simulink model "QubeServo3Pendulum_Workspace"  (R2023a)
settings: Solver=ode4  StartTime=0.0  StopTime=inf  FixedStep=1/1000  RelTol=1e-3  EnableMultiTasking=on
model workspace (MAT data in the model file):
  Jp = 0.000133128
  Jr = 0.000228791666667
  Jr_stall = 1
  Jt = 1.31452806e-08
  Lp = 0.129
  Rm = 7.5
  bp = 3e-05
  bpp = 5e-05
  bpr = 0.000425
  br = 2.15e-05
  br_stall = 100
  brp = 0
  brr = 0.0005
  g = 9.81
  km = 0.0422
  kr = 0.0005
  kt = 0.0422
  l = 0.0645
  mp = 0.024
  mr = 0.095
  r = 0.085
libraries: quarc_library x6, simulink x6, simulink_extras x2
settings Model: SimulationMode=external  ExtModeTrigDuration=10000  Creator=mbohra  LastModifiedBy=mbohra
settings SolverCC: AlgebraicLoopSolver=TrustRegion  PositivePriorityOrder=on
settings DataIOCC: ReturnWorkspaceOutputs=off
settings OptimizationCC: ReuseModelBlockBuffer=off
settings DebuggingCC: UnconnectedInputMsg=warning  UnconnectedOutputMsg=warning  UnconnectedLineMsg=warning  ArithmeticOperatorsInVariantConditions=warning
settings ModelReferenceCC: EnableRefExpFcnMdlSchedulingChecks=on
settings SFSimCC: SimUseLocalCustomCode=off  CustomCodeUndefinedFunction=UseInterfaceOnly
settings RTWCC: Description=QUARC Win64 Target Using Toolchain  SystemTargetFile=quarc_win64.tlc  TemplateMakefile=quarc_default_tmf  RTWUseLocalCustomCode=off  Toolchain=QUARC win64 | nmake (64-bit Windows)  BuildConfiguration=Faster Runs  DLArmComputeVersion=19.05
settings CodeAppCC: StateflowObjectComments=on
settings STFCustomTargetCC: SystemTargetFile=quarc_win64.tlc
settings GRTTargetCC: ParMdlRefBuildCompliant=off  CompOptLevelCompliant=off  CombineOutputUpdateFcns=off  MatFileLogging=off  CPPClassGenCompliant=off  GRTInterface=on  ExtMode=on  ExtModeMexFile=quarc_comm
settings ConfigComp: CovMetricSettings=dswe

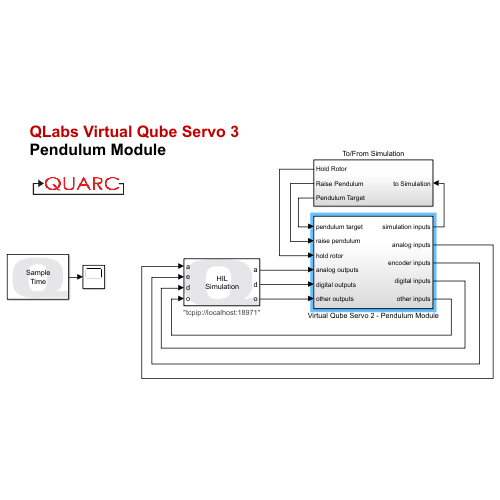
[thumbnail: Simulink's stored preview of the top-level diagram]
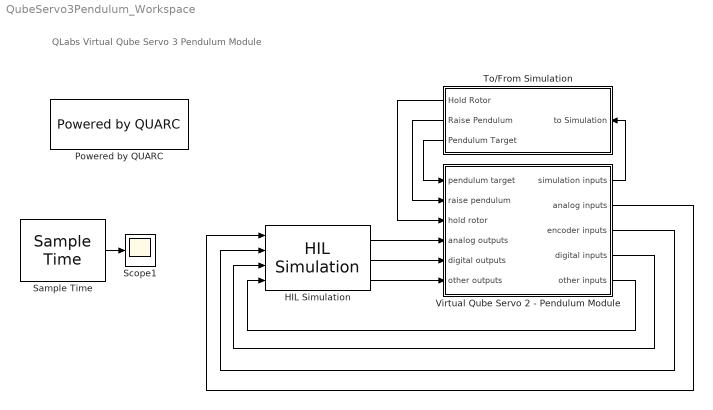
== system QubeServo3Pendulum_Workspace ==
  note: QLabs Virtual Qube Servo 3
      | Pendulum Module
  HIL Simulation : quarc_library/Data Acquisition/Generic/Configuration/HIL Simulation  uri_source=Specify via dialog (do not evaluate)  uri=tcpip://localhost:18971  board_type=qube_servo3_usb  board_id=0  sample_time=qc_get_step_size  active=on  num_clocks=1  num_interrupts=0  num_analog_inputs=1  num_analog_outputs=1  initial_analog=[]  num_digital_io=0  num_digital_inputs=3  num_digital_outputs=1  initial_digital=[]  num_encoder_inputs=2  num_pwm_outputs=0  initial_pwm=[]  other_inputs=[14000]  other_outputs=[11000:11002]  initial_other=[]  integer_get_property_codes=[]  double_get_property_codes=[]  string_get_property_codes=[]  integer_set_property_codes=[]  double_set_property_codes=[]  string_set_property_codes=[]  initial_integer_properties=0  initial_double_properties=0  max_string_property=80  use_variable_size_strings=off
      settings: AttributesFormatString="\"tcpip://localhost:18971\""  SourceProductName=QUARC Targets
  Powered by QUARC : quarc_library/Logos/Powered by QUARC
  Sample Time : quarc_library/Sources/Time/Sample Time  Priority=-99  sample_time=qc_get_step_size
  Scope1 : Scope
  To/From Simulation : Subsystem
  Virtual Qube Servo 2 - Pendulum Module : Subsystem
  wires:
  Sample Time/1 -> Scope1/1
  Virtual Qube Servo 2 - Pendulum Module/1(simulation inputs) -> To/From Simulation/1(to Simulation)
  HIL Simulation/1 -> Virtual Qube Servo 2 - Pendulum Module/4(analog outputs)
  HIL Simulation/2 -> Virtual Qube Servo 2 - Pendulum Module/5(digital outputs)
  Virtual Qube Servo 2 - Pendulum Module/2(analog inputs) -> HIL Simulation/1
  Virtual Qube Servo 2 - Pendulum Module/5(other inputs) -> HIL Simulation/4
  Virtual Qube Servo 2 - Pendulum Module/3(encoder inputs) -> HIL Simulation/2
  Virtual Qube Servo 2 - Pendulum Module/4(digital inputs) -> HIL Simulation/3
  To/From Simulation/2(Raise Pendulum) -> Virtual Qube Servo 2 - Pendulum Module/2(raise pendulum)
  To/From Simulation/1(Hold Rotor) -> Virtual Qube Servo 2 - Pendulum Module/3(hold rotor)
  HIL Simulation/3 -> Virtual Qube Servo 2 - Pendulum Module/6(other outputs)
  To/From Simulation/3(Pendulum Target) -> Virtual Qube Servo 2 - Pendulum Module/1(pendulum target)

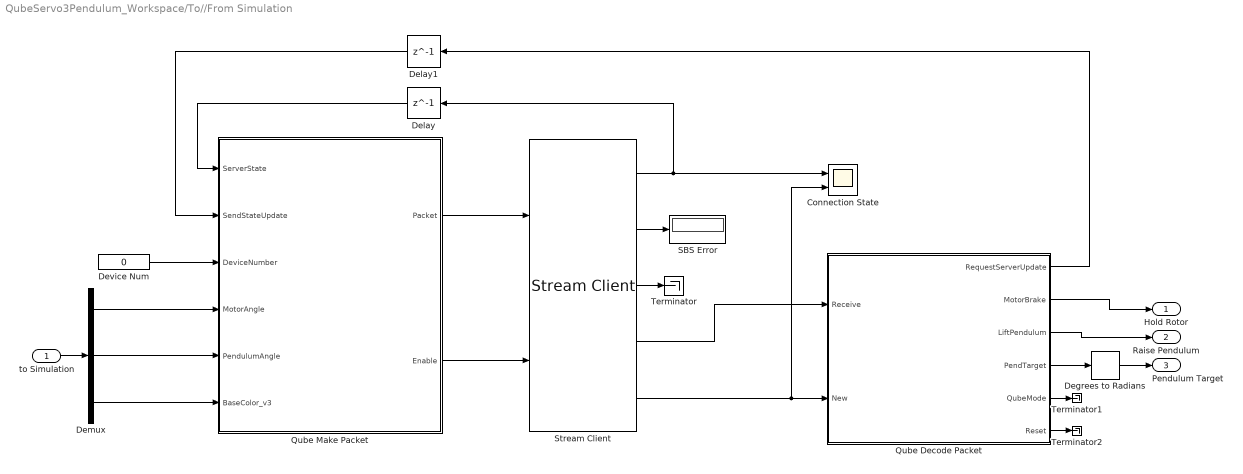
== system QubeServo3Pendulum_Workspace/To//From Simulation ==
  to Simulation : Inport
  "Connection State " : Scope  NumInputPorts=2
  Degrees to Radians : simulink_extras/Transformations/Degrees to Radians
  Delay : Delay  DelayLength=1
  Delay1 : Delay  DelayLength=1
  Demux : Demux  Outputs=[1,1,3]
  Device Num : Constant  Value=0
  Qube Decode Packet : MATLAB Function  TreatAsAtomicUnit=on
  Qube Make Packet : MATLAB Function  TreatAsAtomicUnit=on
  SBS Error : Display
  Stream Client : quarc_library/Communications/Basic/Stream Client  uri_source=Specify via dialog (do not evaluate)  uri=tcpip://localhost:18000?nagle='off'  send_buffer_size=65537  receive_buffer_size=65537  byte_order=little endian (Intel - LSB first)  optimization=Minimum latency  send_options=Send all data  receive_options=Receive all data  default_value=[0]  sample_time=qc_get_step_size  active=off  implementation=Use blocking I/O in a separate thread  send_fifo_size=3  receive_fifo_size=3  send_priority=0  receive_priority=0  send_dimensions=on  receive_dimensions=on  max_dimensions=65537  data_type=uint8  type_expr=BusObject
      settings: AttributesFormatString="\"tcpip://localhost:18000?nagle='off'\""
  Terminator : Terminator
  Terminator1 : Terminator
  Terminator2 : Terminator
  Hold Rotor : Outport  VectorParamsAs1DForOutWhenUnconnected=off
  Raise Pendulum : Outport  Port=2  VectorParamsAs1DForOutWhenUnconnected=off
  Pendulum Target : Outport  Port=3  VectorParamsAs1DForOutWhenUnconnected=off
  wires:
  Qube Make Packet/1(Packet) -> Stream Client/1
  Qube Make Packet/2(Enable) -> Stream Client/2
  Stream Client/2 -> SBS Error/1
  Demux/3 -> Qube Make Packet/6(BaseColor_v3)
  Qube Decode Packet/3(LiftPendulum) -> Raise Pendulum/1
  Delay/1 -> Qube Make Packet/1(ServerState)
  Stream Client/1 -> Delay/1, "Connection State "/1
  Stream Client/3 -> Terminator/1
  Qube Decode Packet/2(MotorBrake) -> Hold Rotor/1
  Delay1/1 -> Qube Make Packet/2(SendStateUpdate)
  Device Num/1 -> Qube Make Packet/3(DeviceNumber)
  Stream Client/5 -> "Connection State "/2, Qube Decode Packet/2(New)
  Demux/1 -> Qube Make Packet/4(MotorAngle)
  Qube Decode Packet/1(RequestServerUpdate) -> Delay1/1
  Stream Client/4 -> Qube Decode Packet/1(Receive)
  Demux/2 -> Qube Make Packet/5(PendulumAngle)
  to Simulation/1 -> Demux/1
  Qube Decode Packet/5(QubeMode) -> Terminator1/1
  Qube Decode Packet/6(Reset) -> Terminator2/1
  Qube Decode Packet/4(PendTarget) -> Degrees to Radians/1
  Degrees to Radians/1 -> Pendulum Target/1

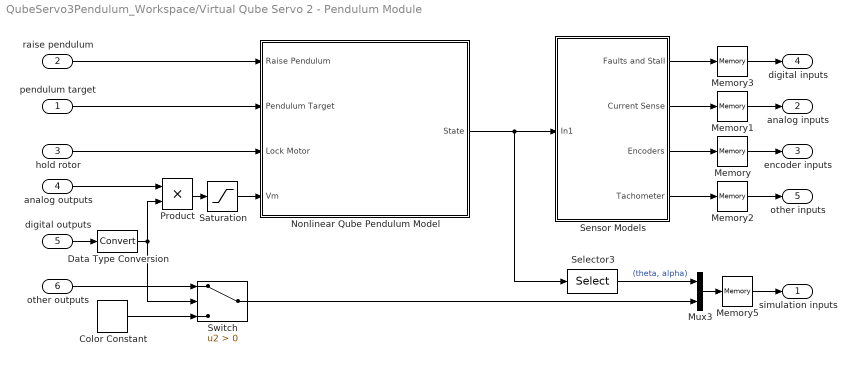
== system QubeServo3Pendulum_Workspace/Virtual Qube Servo 2 - Pendulum Module ==
  pendulum target : Inport
  raise pendulum : Inport  Port=2
  hold rotor : Inport  Port=3
  analog outputs : Inport  Port=4
  digital outputs : Inport  Port=5
  other outputs : Inport  Port=6
  Color Constant : quarc_library/Sources/Signals/Color Constant  color=[1 0 0]
      settings: SourceProductName=QUARC Targets
  Data Type Conversion : DataTypeConversion  SaturateOnIntegerOverflow=off  RndMeth=Floor
  Memory : Memory  InitialCondition=[0 0]  InheritSampleTime=on
  Memory1 : Memory
  Memory2 : Memory
  Memory3 : Memory  InitialCondition=[0 0 0]
  Memory5 : Memory  InitialCondition=[0 0 1 0 0]
  Mux3 : Mux  Inputs=2
  Nonlinear Qube Pendulum Model : Subsystem
  Product : Product
  Saturation : Saturate  UpperLimit=15  LowerLimit=-15
  Selector3 : Selector  InputPortWidth=5  IndexOptions=Index vector (dialog)  Indices=1:2  OutputSizes=1
  Sensor Models : Subsystem
  Switch : Switch  Criteria=u2 > Threshold  SaturateOnIntegerOverflow=off  InputSameDT=off
  simulation inputs : Outport  VectorParamsAs1DForOutWhenUnconnected=off
  analog inputs : Outport  Port=2  VectorParamsAs1DForOutWhenUnconnected=off
  encoder inputs : Outport  Port=3  VectorParamsAs1DForOutWhenUnconnected=off
  digital inputs : Outport  Port=4  VectorParamsAs1DForOutWhenUnconnected=off
  other inputs : Outport  Port=5  VectorParamsAs1DForOutWhenUnconnected=off
  wires:
  analog outputs/1 -> Product/1
  digital outputs/1 -> Data Type Conversion/1
  other outputs/1 -> Switch/1
  Data Type Conversion/1 -> Switch/2, Product/2
  Memory/1 -> encoder inputs/1
  Memory1/1 -> analog inputs/1
  Memory2/1 -> other inputs/1
  Memory3/1 -> digital inputs/1
  Product/1 -> Saturation/1
  Selector3/1 -> Mux3/1  "(theta, alpha)"
  Mux3/1 -> Memory5/1
  Nonlinear Qube Pendulum Model/1(State) -> Selector3/1, Sensor Models/1(In1)
  Memory5/1 -> simulation inputs/1
  raise pendulum/1 -> Nonlinear Qube Pendulum Model/1(Raise Pendulum)
  Saturation/1 -> Nonlinear Qube Pendulum Model/4(Vm)
  hold rotor/1 -> Nonlinear Qube Pendulum Model/3(Lock Motor)
  pendulum target/1 -> Nonlinear Qube Pendulum Model/2(Pendulum Target)
  Color Constant/1 -> Switch/3
  Switch/1 -> Mux3/2
  Sensor Models/1(Faults and Stall) -> Memory3/1
  Sensor Models/2(Current Sense) -> Memory1/1
  Sensor Models/3(Encoders) -> Memory/1
  Sensor Models/4(Tachometer) -> Memory2/1

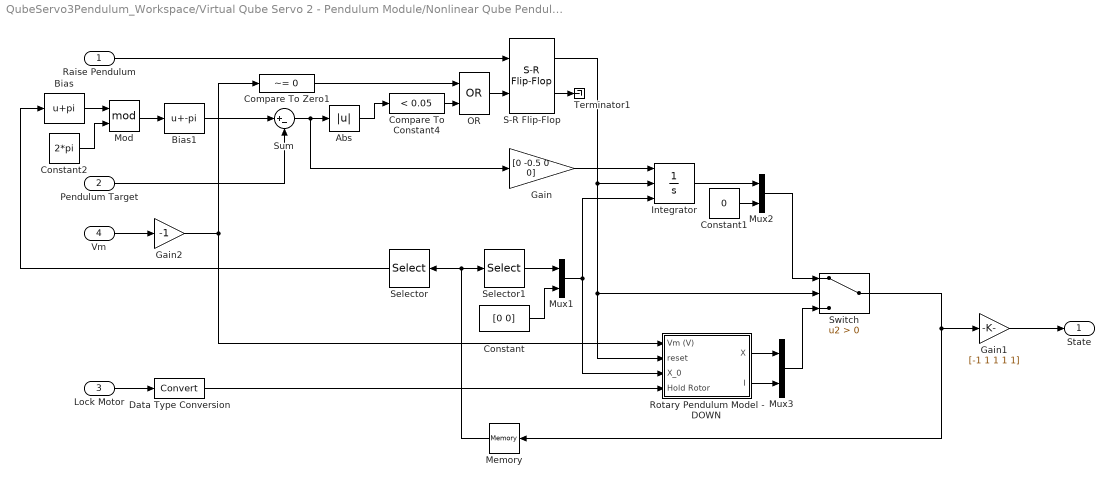
== system QubeServo3Pendulum_Workspace/Virtual Qube Servo 2 - Pendulum Module/Nonlinear Qube Pendulum Model ==
  Raise Pendulum : Inport
  Pendulum Target : Inport  Port=2
  Lock Motor : Inport  Port=3
  Vm : Inport  Port=4
  Abs : Abs  SaturateOnIntegerOverflow=off
  Bias : Bias  Bias=pi  SaturateOnIntegerOverflow=off
  Bias1 : Bias  Bias=-pi  SaturateOnIntegerOverflow=off
  Compare To Constant4 : simulink/Logic and Bit Operations/Compare To Constant  relop=<  const=0.05  OutDataTypeStr=boolean
  Compare To Zero1 : simulink/Logic and Bit Operations/Compare To Zero  relop=~=  OutDataTypeStr=boolean
  Constant : Constant  Value=[0 0]
  Constant1 : Constant  Value=0
  Constant2 : Constant  Value=2*pi
  Data Type Conversion : DataTypeConversion  SaturateOnIntegerOverflow=off  RndMeth=Floor
  Gain : Gain  Gain=[0 -0.5 0 0]
  Gain1 : Gain  Gain=[-1 1 1 1 1]
  Gain2 : Gain  Gain=-1
  Integrator : Integrator  ExternalReset=rising  InitialConditionSource=external
  Memory : Memory
  Mod : Math  Operator=mod  SignedPower=on
  Mux1 : Mux  Inputs=2
  Mux2 : Mux  Inputs=2
  Mux3 : Mux  Inputs=2
  OR : Logic  Operator=OR  IconShape=distinctive  AllPortsSameDT=off  OutDataTypeStr=boolean
  Rotary Pendulum Model - DOWN : Subsystem
  S-R Flip-Flop : simulink_extras/Flip Flops/S-R Flip-Flop  initial_condition=0
  Selector : Selector  InputPortWidth=5  IndexOptions=Index vector (dialog)  Indices=[2]  OutputSizes=1
  Selector1 : Selector  InputPortWidth=5  IndexOptions=Index vector (dialog)  Indices=[1 2]  OutputSizes=1
  Sum : Sum  Inputs=|+-
  Switch : Switch  Criteria=u2 > Threshold  SaturateOnIntegerOverflow=off  InputSameDT=off
  Terminator1 : Terminator
  State : Outport  VectorParamsAs1DForOutWhenUnconnected=off
  wires:
  S-R Flip-Flop/2 -> Terminator1/1
  Compare To Constant4/1 -> OR/2
  Compare To Zero1/1 -> OR/1
  OR/1 -> S-R Flip-Flop/2
  Raise Pendulum/1 -> S-R Flip-Flop/1
  S-R Flip-Flop/1 -> Integrator/2, Switch/2, Rotary Pendulum Model - DOWN/2(reset)
  Abs/1 -> Compare To Constant4/1
  Lock Motor/1 -> Data Type Conversion/1
  Memory/1 -> Selector1/1, Selector/1
  Switch/1 -> Memory/1, Gain1/1
  Selector1/1 -> Mux1/1
  Constant/1 -> Mux1/2
  Gain/1 -> Integrator/1
  Integrator/1 -> Mux2/1
  Mux2/1 -> Switch/1
  Constant1/1 -> Mux2/2
  Pendulum Target/1 -> Sum/2
  Constant2/1 -> Mod/2
  Selector/1 -> Bias/1
  Mod/1 -> Bias1/1
  Sum/1 -> Gain/1, Abs/1
  Bias/1 -> Mod/1
  Bias1/1 -> Sum/1
  Vm/1 -> Gain2/1
  Mux1/1 -> Integrator/3, Rotary Pendulum Model - DOWN/3(X_0)
  Rotary Pendulum Model - DOWN/1(X) -> Mux3/1
  Rotary Pendulum Model - DOWN/2(I) -> Mux3/2
  Mux3/1 -> Switch/3
  Gain1/1 -> State/1
  Gain2/1 -> Rotary Pendulum Model - DOWN/1(Vm (V)), Compare To Zero1/1
  Data Type Conversion/1 -> Rotary Pendulum Model - DOWN/4(Hold Rotor)

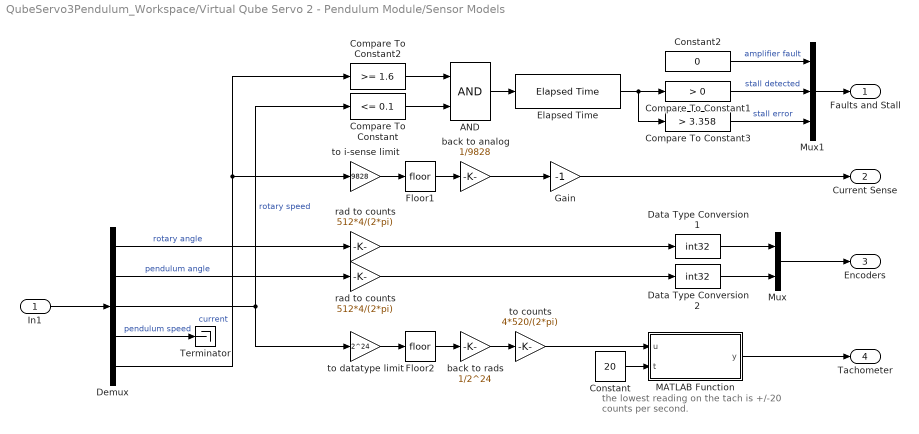
== system QubeServo3Pendulum_Workspace/Virtual Qube Servo 2 - Pendulum Module/Sensor Models ==
  note: the lowest reading on the tach
      | is +/-20 counts per second.
  In1 : Inport
  AND : Logic  AllPortsSameDT=off  OutDataTypeStr=boolean
  Compare To Constant : simulink/Logic and Bit Operations/Compare To Constant  relop=<=  const=0.1  OutDataTypeStr=boolean
  Compare To Constant1 : simulink/Logic and Bit Operations/Compare To Constant  relop=>  const=0  OutDataTypeStr=boolean
  Compare To Constant2 : simulink/Logic and Bit Operations/Compare To Constant  relop=>=  const=1.6  OutDataTypeStr=boolean
  Compare To Constant3 : simulink/Logic and Bit Operations/Compare To Constant  relop=>  const=3.358  OutDataTypeStr=boolean
  Constant : Constant  Value=20
  Constant2 : Constant  Value=0  OutDataTypeStr=Inherit: Inherit via back propagation
  Data Type Conversion1 : DataTypeConversion  OutDataTypeStr=int32  SaturateOnIntegerOverflow=off  RndMeth=Floor
  Data Type Conversion2 : DataTypeConversion  OutDataTypeStr=int32  SaturateOnIntegerOverflow=off  RndMeth=Floor
  Demux : Demux  Outputs=5
  Elapsed Time : quarc_library/Advanced/Timing/Elapsed Time  start_src=on  sample_time=-1
      settings: SourceProductName=QUARC Targets
  Floor1 : Rounding
  Floor2 : Rounding
  Gain : Gain  Gain=-1
  MATLAB Function : MATLAB Function  TreatAsAtomicUnit=on
  Mux : Mux  Inputs=2
  Mux1 : Mux  Inputs=3
  Terminator : Terminator
  back to rads : Gain  Gain=1/2^24
  back to analog : Gain  Gain=1/9828
  rad to counts : Gain  Gain=512*4/(2*pi)
  "rad to counts " : Gain  Gain=512*4/(2*pi)
  to counts : Gain  Gain=4*520/(2*pi)
  to datatype limit : Gain  Gain=2^24
  to i-sense limit : Gain  Gain=9828
  Faults and Stall : Outport  VectorParamsAs1DForOutWhenUnconnected=off
  Current Sense : Outport  Port=2  VectorParamsAs1DForOutWhenUnconnected=off
  Encoders : Outport  Port=3  VectorParamsAs1DForOutWhenUnconnected=off
  Tachometer : Outport  Port=4  VectorParamsAs1DForOutWhenUnconnected=off
  wires:
  Gain/1 -> Current Sense/1
  Compare To Constant3/1 -> Mux1/3  "stall error"
  to i-sense limit/1 -> Floor1/1
  to datatype limit/1 -> Floor2/1
  Floor1/1 -> back to analog/1
  Compare To Constant2/1 -> AND/1
  back to rads/1 -> to counts/1
  AND/1 -> Elapsed Time/1
  Demux/1 -> rad to counts/1  "rotary angle"
  Constant2/1 -> Mux1/1  "amplifier fault"
  Floor2/1 -> back to rads/1
  rad to counts/1 -> Data Type Conversion1/1
  back to analog/1 -> Gain/1
  to counts/1 -> MATLAB Function/1(u)
  In1/1 -> Demux/1
  Demux/4 -> Terminator/1  "pendulum speed"
  Constant/1 -> MATLAB Function/2(t)
  Data Type Conversion1/1 -> Mux/1
  Demux/3 -> to datatype limit/1, Compare To Constant/1  "rotary speed"
  Elapsed Time/1 -> Compare To Constant1/1, Compare To Constant3/1
  Compare To Constant/1 -> AND/2
  Demux/2 -> "rad to counts "/1  "pendulum angle"
  Data Type Conversion2/1 -> Mux/2
  "rad to counts "/1 -> Data Type Conversion2/1
  Demux/5 -> Compare To Constant2/1, to i-sense limit/1  "current"
  Compare To Constant1/1 -> Mux1/2  "stall detected"
  MATLAB Function/1(y) -> Tachometer/1
  Mux/1 -> Encoders/1
  Mux1/1 -> Faults and Stall/1

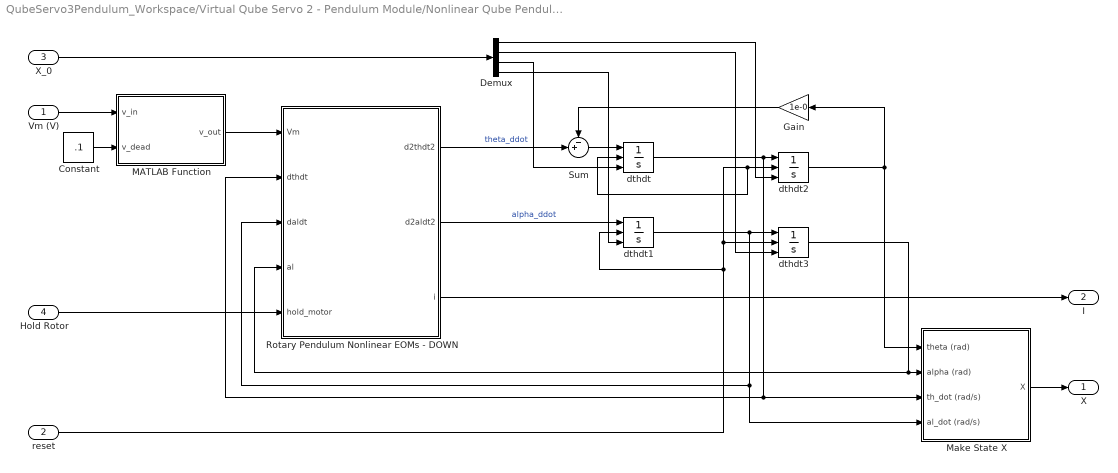
== system QubeServo3Pendulum_Workspace/Virtual Qube Servo 2 - Pendulum Module/Nonlinear Qube Pendulum Model/Rotary Pendulum Model - DOWN ==
  Vm (V) : Inport
  reset : Inport  Port=2
  X_0 : Inport  Port=3
  Hold Rotor : Inport  Port=4
  Constant : Constant  Value=.1
  Demux : Demux
  Gain : Gain  Gain=1e-0
  MATLAB Function : MATLAB Function  TreatAsAtomicUnit=on
  Make State X : Subsystem
  Rotary Pendulum Nonlinear EOMs - DOWN : MATLAB Function  TreatAsAtomicUnit=on
  Sum : Sum  Inputs=-+|
  dthdt : Integrator  ExternalReset=falling  InitialConditionSource=external
  dthdt1 : Integrator  ExternalReset=falling  InitialConditionSource=external
  dthdt2 : Integrator  ExternalReset=falling  InitialConditionSource=external  LimitOutput=on  UpperSaturationLimit=pi*135/180  LowerSaturationLimit=-pi*135/180
  dthdt3 : Integrator  ExternalReset=falling  InitialConditionSource=external
  X : Outport  VectorParamsAs1DForOutWhenUnconnected=off
  I : Outport  Port=2  VectorParamsAs1DForOutWhenUnconnected=off
  wires:
  dthdt3/1 -> Make State X/2(alpha (rad)), Rotary Pendulum Nonlinear EOMs - DOWN/4(al)
  Rotary Pendulum Nonlinear EOMs - DOWN/2(d2aldt2) -> dthdt1/1  "alpha_ddot"
  Make State X/1(X) -> X/1
  dthdt1/1 -> Make State X/4(al_dot (rad/s)), Rotary Pendulum Nonlinear EOMs - DOWN/3(daldt), dthdt3/1
  dthdt2/1 -> Gain/1, Make State X/1(theta (rad))
  dthdt/1 -> Rotary Pendulum Nonlinear EOMs - DOWN/2(dthdt), Make State X/3(th_dot (rad/s)), dthdt2/1
  reset/1 -> dthdt3/2, dthdt/2, dthdt2/2, dthdt1/2
  X_0/1 -> Demux/1
  Demux/1 -> dthdt2/3
  Demux/2 -> dthdt3/3
  Demux/3 -> dthdt/3
  Demux/4 -> dthdt1/3
  Rotary Pendulum Nonlinear EOMs - DOWN/1(d2thdt2) -> Sum/2  "theta_ddot"
  Sum/1 -> dthdt/1
  Gain/1 -> Sum/1
  MATLAB Function/1(v_out) -> Rotary Pendulum Nonlinear EOMs - DOWN/1(Vm)
  Vm (V)/1 -> MATLAB Function/1(v_in)
  Constant/1 -> MATLAB Function/2(v_dead)
  Rotary Pendulum Nonlinear EOMs - DOWN/3(i) -> I/1
  Hold Rotor/1 -> Rotary Pendulum Nonlinear EOMs - DOWN/5(hold_motor)

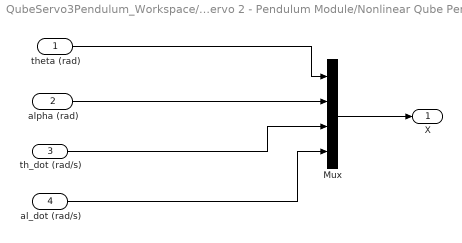
== system QubeServo3Pendulum_Workspace/Virtual Qube Servo 2 - Pendulum Module/Nonlinear Qube Pendulum Model/Rotary Pendulum Model - DOWN/Make State X ==
  theta (rad) : Inport
  alpha (rad) : Inport  Port=2
  th_dot (rad/s) : Inport  Port=3
  al_dot (rad/s) : Inport  Port=4
  Mux : Mux
  X : Outport  VectorParamsAs1DForOutWhenUnconnected=off
  wires:
  alpha (rad)/1 -> Mux/2
  al_dot (rad/s)/1 -> Mux/4
  th_dot (rad/s)/1 -> Mux/3
  Mux/1 -> X/1
  theta (rad)/1 -> Mux/1

== matlab function QubeServo3Pendulum_Workspace/Virtual Qube Servo 2 - Pendulum Module/Sensor Models/MATLAB Function ==
  data: u input; y output; t input
function y = tach_model(u, t)

y = u;

if (u >= 0)&&(u < t)
    y = t;
elseif (u < 0)&&(u > -t)
    y = -t;
end

== matlab function QubeServo3Pendulum_Workspace/To//From Simulation/Qube Decode Packet ==
  data: Receive input size=65537; RequestServerUpdate output; New input; MotorBrake output; LiftPendulum output; PendTarget output; QubeMode output; Reset output
function [RequestServerUpdate, MotorBrake, LiftPendulum, PendTarget, QubeMode, Reset] = QubeDecodePacket(Receive, New)

%% Setup

persistent iMotorBrake;
persistent iQubeMode;
persistent iPendTarget;

if isempty(iMotorBrake)
    iMotorBrake = uint8(0);
    iQubeMode = uint8(1);
    iPendTarget = uint8(180);
end

% Need to assign outputs here even though they are reassigned at the end
% since matlab can't determine the signal widths
MotorBrake = false;
LiftPendulum = false;
QubeMode = uint8(0);
PendTarget = 180;
Reset = 0;
RequestServerUpdate = 0;

PacketSize = length(Receive);

% Packet > 0, new data, and magic number in first index
if ((PacketSize > 0) && (New == 1) && (Receive(1) == uint8(123)))
    
    %skip magic number
    Index = int32(2);
    
    while(Index <= PacketSize)
       
        %% Get container details
        ContainerSize = typecast(uint8(flip(Receive(Index:Index+3))), 'int32');
        DeviceID = typecast(uint8(flip(Receive(Index+4:Index+7))), 'int32');
        DeviceNum = typecast(uint8(flip(Receive(Index+8:Index+11))), 'int32');
        DeviceFunction = uint8(Receive(Index+12));
        PayloadStart = Index+13;
        PayloadEnd = Index+ContainerSize-1;
        
        %% Pass container to appropriate decoding function
        if (DeviceID == 61) %is this a Qube2 container?
            
            if (DeviceFunction == 11) %UE4 State Response
                iMotorBrake = uint8(Receive(PayloadStart));
                RequestServerUpdate = 1;
            elseif (DeviceFunction == 13) %Mode Response
                iQubeMode = uint8(Receive(PayloadStart));
            elseif (DeviceFunction == 100) %Lift Pendulum Event
                LiftPendulum = true; 
                iPendTarget = uint8(Receive(PayloadStart));
            end
        
        elseif (DeviceID == 1001) %Simulink notification
            if (DeviceFunction == 200) %Reset button
                Reset = 1;
            end
        end
        
        
        
        %% Process next container if any data is left.
        Index = Index+ContainerSize;
    end


end

MotorBrake = (iMotorBrake > 0);
QubeMode = iQubeMode;
PendTarget = double(iPendTarget);

== matlab function QubeServo3Pendulum_Workspace/Virtual Qube Servo 2 - Pendulum Module/Nonlinear Qube Pendulum Model/Rotary Pendulum Model - DOWN/MATLAB Function ==
  data: v_in input; v_out output; v_dead input
function v_out = fcn(v_in, v_dead)
v_out = v_in;
if abs(v_in) < v_dead
    v_out = 0;
end
end

== matlab function QubeServo3Pendulum_Workspace/To//From Simulation/Qube Make Packet ==
  settings: updateMethod=DISCRETE  sampleTime=qc_get_step_size
  data: Packet output size=65537; ServerState input; SendStateUpdate input; Enable output; DeviceNumber input; MotorAngle input; PendulumAngle input; BaseColor_v3 input
function [Packet,Enable] = QubeMakePacket(ServerState, SendStateUpdate, DeviceNumber, MotorAngle, PendulumAngle, BaseColor_v3) 

% Be sure to set the maximum signal size of the variable size Packet port 
% in Simulink->Edit Data of the editor window.  Size should be 65537 or
% larger to ensure that the stream server generates a 4 byte packet size.

%% Setup
persistent LastServerState;
%persistent ModeDataAge;

if isempty(LastServerState)
    LastServerState = uint8(0);
    %ModeDataAge = 0;
end

Enable = 0;
Packet = uint8([]);

%% On connection
if ((ServerState == 2) && (LastServerState ~= 2))
    Packet = Qube3MakeCommandStateContainer(DeviceNumber, MotorAngle, PendulumAngle, BaseColor_v3); 
    Packet = [Packet; Qube3MakeModeRequestContainer(DeviceNumber)];
end

%% Send new State Container
% Previous state processed, send a new one
if (SendStateUpdate)
    Packet = Qube3MakeCommandStateContainer(DeviceNumber, MotorAngle, PendulumAngle, BaseColor_v3);
end

%% Transmit
% If we have data to send, enable the transmit
PacketLength = length(Packet);

if (PacketLength > 0)
    % Add magic byte.  This is just for error handling and isn't typically
    % required in simulink, but useful in lower-level languages like Python
    Packet = [uint8(123); Packet];
    
    Enable = 1; 
end


LastServerState = ServerState;

== matlab function QubeServo3Pendulum_Workspace/Virtual Qube Servo 2 - Pendulum Module/Nonlinear Qube Pendulum Model/Rotary Pendulum Model - DOWN/Rotary Pendulum Nonlinear EOMs - DOWN ==
  data: Vm input size=1; d2thdt2 output size=1; d2aldt2 output size=1; dthdt input size=1; daldt input size=1; Jp parameter; Jr parameter; l parameter; mp parameter; br parameter; bp parameter; r parameter; kt parameter; km parameter; Rm parameter; al input size=1; g parameter; i output; Jr_stall parameter; br_stall parameter; hold_motor input
function [d2thdt2,d2aldt2,i] = pen_nonlin_eoms(Vm, dthdt, daldt, Jp, Jr, l, mp, br, bp, r, kt, km, Rm, al, g, Jr_stall, br_stall, hold_motor)

if hold_motor
    rotor_inertia = Jr_stall;
    rotor_damping = br_stall;
else
    rotor_inertia = Jr;
    rotor_damping = br;
end
% Convert voltage to torque input
i = (Vm - km*dthdt)/Rm;
tau=kt*i;
% Denominator
Jt = rotor_inertia*Jp + Jp^2*sin(al)^2 - mp^2*r^2*l^2*cos(al)^2;
% Nonlinear equations of motion for generic rotary pendulum (i.e. furuta)
% Terms from EOM solving
term1 = tau - rotor_damping*dthdt + 2*Jp*sin(al)*cos(al)*dthdt*daldt + mp*r*l*sin(al)*daldt^2;
term2 = -bp*daldt - Jp*sin(al)*cos(al)*daldt^2 - mp*g*l*sin(al);
% Torque to rotary arm position)
d2thdt2 = 1/Jt*( Jp*term1 - mp*r*l*cos(al)*term2);
% Torque to pendulum angle position
d2aldt2 = 1/Jt*(-mp*r*l*cos(al)*term1 + (rotor_inertia+Jp*sin(al)^2)*term2);
